simulink model "PubIfDecisionTOS_MDL"  (R2020b)
settings: configuration reference "DspaceConfig" (kept outside this file)
PostLoadFcn:
  | if any(exist('dsrtsu_mdlpostloadfcn', 'file') ~= 0), dsrtsu_mdlpostloadfcn('Execute', bdroot); end
InitFcn:
  | , if any(exist('dsmpb_private', 'file') ~= 0), dsmpb_private('dsmpb_mdlclblib', 'Init', bdroot); end,
undefined symbols (not defined in the file or in its folder): C_TOS_ACCEgoRAxletoFbumplength_m, C_TOS_ACCTargetFront_Flag, C_TOS_AEBJAPedObjDxThre_Val, C_TOS_AEBJAPedObjDyThre_Val, C_TOS_AEBJATargetSize_Val, C_TOS_AEBJAVehObjDxThre_Val, C_TOS_AEBJAVehObjDyThre_Val, C_TOS_AEBJuncPedTargetSize_Val, C_TOS_AEBLatObjDxThre_Val, C_TOS_AEBLatPedDyThre_Val, C_TOS_AEBLatTargetSize_Val, C_TOS_AEBLongTargetInEgoFront_Flag, C_TOS_axAbsGround_Parameter, C_TOS_CameraConfirmedFlag, C_TOS_CNsubjWidth, C_TOS_CurrentLaneCoreMinWidth_Val, C_TOS_CutInProb_Val_Zero, C_TOS_CutOutProb_Val_Zero, C_TOS_D2R_Val, C_TOS_DefaultValueObjectToCenterLine_dy, C_TOS_EgoCarWidth_Val, C_TOS_EgoDxRefPoint_m, C_TOS_EgoRAxletoFbumplength_m, C_TOS_HalfWidthVehicle_Con, C_TOS_HWA_CurrentLaneFlag, C_TOS_HWA_LeftLaneFlag, C_TOS_HWA_MovingDir_Vaild, C_TOS_HWA_MovState_Vaild, C_TOS_HWA_RightLaneFlag, C_TOS_LaneLineCourseErrorFront, C_TOS_LaneLineCourseErrorRear, C_TOS_MotorbikeDefaultWidth_m, C_TOS_NumberOfEffectiveTargets, C_TOS_Obj_Age_Val, C_TOS_Objdx_Constraint_Val, C_TOS_ObjectDefaultWidth_m, C_TOS_ObjInCurrentLane_Val, C_TOS_ObjInCurrentLaneValid, C_TOS_ObjInLeftLaneValid, C_TOS_ObjInRightLaneValid, C_TOS_ObjNotInCurrentLane_Val, C_TOS_ObjNotREElementType, C_TOS_ObjPredictDis_dy_ConstantVal_Zeros, C_TOS_ObjToCenterLine_ConstantVal_Zeros, C_TOS_OFMObjIDInvilad_Val, C_TOS_PIL_LatDisCons_Val_zero, C_TOS_PIL_ObjectCutInFlag_b, C_TOS_PIL_ObjectCutOutFlag_b, C_TOS_PIL_ObjLaneProb_al_Val, C_TOS_PP_ObjFusType_FC_Confirm_b, C_TOS_PP_ObjFusType_FC_FR_Confirm_b, C_TOS_PP_ObjFusType_FR_Confirm_b, C_TOS_RE_80BoolDefault_Val, C_TOS_RE_80Single181Default_Val, C_TOS_RE_80Single255Default_Val, C_TOS_RE_80Uint8Default_Val, C_TOS_RE_D2R, C_TOS_RE_D_180_Val, C_TOS_RE_InvalidObjectID_Val, C_TOS_RE_InvalidTargetChainDir_Val ... (+142)
libraries: simulink x1650, TOS_LIB x361, canfdmsglib x14
(part 2 of 69)

== system PubIfDecisionTOS_MDL/TOS_20201112/TOS_2012080320/Subsystem ==
  TOS_AEBLONOBJ : Inport
  TOS_AEB_JAOBJ : Inport  Port=2
  TOS_AEB_LATOBJ : Inport  Port=3
  Bus Selector : BusSelector  OutputSignals=FusionType,ObjUpdate,ObjectAzimuthAngle,ObjectExistProb,ObjectHight,ObjectID,ObjectIsObstacleProb,ObjectLength,ObjectLengthVar,ObjectLifeCycle,ObjectMeasurementStatus,ObjectMovingOrientationProb,ObjectMovingOrientation,ObjectMovingState,ObjectMovingStateProb,ObjectRCS,ObjectType,ObjectTypeCameraConfirmed,ObjectTypeProb,ObjectWidth,ObjectWidthVar,ObjectYawAngle,ObjectYawAngleVar,ax,axVariance,ay,ayVariance,dx,dxFisrtDetection,dxVariance,dy,dyEgo2Center,dyFisrtDetection,dyObject2Center,dyVariance,dz,vx,vxVariance,vy,vyVariance
  CAN FD Pack : canfdmsglib/CAN FD Pack  CANdbFile=F:\InternalData03_ACC_AEBLog_ELK_LC_LCKie_20200927.dbc  MsgList=(none)  MsgName=TOS_AEBLong  ProtocolMode=CAN FD  MsgIDType=Standard (11-bit identifier)  MsgIdentifier=514  MsgLength=64  Remote=off  BRSSwitch=off  ApplyMinMax=off  SignalInfo={'{'AEBLong_FusionType','24','4','BE','unsigned','Standard','0','1','0','0','15';'AEBLong_ObjUpdate','358','2','BE','unsigned','Standard','0','1','0','0','3';'AEBLong_ObjectAzimuthAngle','231','17','BE','signed','Standard','0','0.0055','0','-360.448','360.4425';'AEBLong_ObjectExistProb','246','10','BE','unsigned','Standard','0','0.000978','0','0','1.0005';'AEBLong_ObjectHight','260','12','BE','unsigned','Standard','0','0.002442','0','0','10';'AEBLong_ObjectID','224','7','BE','unsigned','Standard','0','1','0','0','127';'AEBLong_ObjectIsObstacleProb','278','10','BE','unsigned','Standard','0','0.000978','0','0','1.0005';'AEBLong_ObjectLength','290','14','BE','unsigned','Standard','0','0.0025','0','0','40.9575';'AEBLong_ObjectLengthVar','308','12','BE','unsigned','Standard','0','0.006105','0','0','25';'AEBLong_ObjectLifeCycle','312','8','BE','unsigned','Standard','0','1','0','0','255';'AEBLong_ObjectMeasurementStatus','59','1','BE','unsigned','Standard','0','1','0','0','1';'AEBLong_ObjectMovingOrientProb','334','10','BE','unsigned','Standard','0','0.000978','0','0','1.0005';'AEBLong_ObjectMovingOrientation','104','4','BE','unsigned','Standard','0','1','0','0','15';'AEBLong_ObjectMovingState','120','4','BE','unsigned','Standard','0','1','0','0','15';'AEBLong_ObjectMovingStateProb','350','10','BE','unsigned','Standard','0','0.000978','0','0','1.0005';'AEBLong_ObjectRCS','58','1','BE','unsigned','Standard','0','1','0','0','1';'AEBLong_ObjectType','152','4','BE','unsigned','Standard','0','1','0','0','15';'AEBLong_ObjectTypeCameraConf','57','1','BE','unsigned','Standard','0','1','0','0','1';'AEBLong_ObjectTypeProb','382','10','BE','unsigned','Standard','0','0.000978','0','0','1.0005';'AEBLong_ObjectWidth','396','12','BE','unsigned','Standard','0','0.005','0','0','20.475';'AEBLong_ObjectWidthVar','412','12','BE','unsigned','Standard','0','0.006105','0','0','25';'AEBLong_ObjectYawAngle','439','17','BE','signed','Standard','0','0.0055','0','-360.448','360.4425';'AEBLong_ObjectYawAngleVar','452','12','BE','unsigned','Standard','0','0.006105','0','0','25';'AEBLong_ax','8','16','BE','signed','Standard','0','0.001','0','-32.768','32.767';'AEBLong_axVariance','28','12','BE','unsigned','Standard','0','0.006105','0','0','25';'AEBLong_ay','40','16','BE','signed','Standard','0','0.001','0','-32.768','32.767';'AEBLong_ayVariance','60','12','BE','unsigned','Standard','0','0.006105','0','0','25';'AEBLong_dx','72','16','BE','unsigned','Standard','0','0.0030518','0','0','199.9997';'AEBLong_dxFisrtDetection','88','16','BE','unsigned','Standard','0','0.0030518','0','0','199.9997';'AEBLong_dxVariance','108','12','BE','unsigned','Standard','0','0.006105','0','0','25';'AEBLong_dy','124','12','BE','unsigned','Standard','0','0.009768','0','0','40';'AEBLong_dyEgo2Center','138','14','BE','unsigned','Standard','0','0.0030518','0','0','49.9976';'AEBLong_dyFisrtDetection','156','12','BE','unsigned','Standard','0','0.009768','0','0','40';'AEBLong_dyObject2Center','170','14','BE','unsigned','Standard','0','0.0030518','0','0','49.9976';'AEBLong_dyVariance','188','12','BE','unsigned','Standard','0','0.006105','0','0','25';'AEBLong_dz','204','12','BE','unsigned','Standard','0','0.002442','0','0','10';'AEBLong_vx','472','16','BE','signed','Standard','0','0.006103','0','-199.9831','199.977';'AEBLong_vxVariance','492','12','BE','unsigned','Standard','0','0.006105','0','0','25';'AEBLong_vy','506','14','BE','signed','Standard','0','0.002442','0','-20.0049','20.0024'}
      settings: SourceProductBaseCode=VN  DataFormat=CANdb specified signals
  CAN FD Pack1 : canfdmsglib/CAN FD Pack  CANdbFile=F:\InternalData03_AEB_Lat_JA_20200927.DBC  MsgList=(none)  MsgName=TOS_AEBLarCro_1  ProtocolMode=CAN FD  MsgIDType=Standard (11-bit identifier)  MsgIdentifier=549  MsgLength=64  Remote=off  BRSSwitch=on  ApplyMinMax=off  SignalInfo={'{'AEB_LatCro_FusionType_01','8','7','BE','unsigned','Standard','0','1','0','0','127';'AEB_LatCro_FusionType_02','56','7','BE','unsigned','Standard','0','1','0','0','127';'AEB_LatCro_FusionType_03','96','7','BE','unsigned','Standard','0','1','0','0','127';'AEB_LatCro_FusionType_04','136','7','BE','unsigned','Standard','0','1','0','0','127';'AEB_LatCro_FusionType_05','184','7','BE','unsigned','Standard','0','1','0','0','127';'AEB_LatCro_FusionType_06','224','7','BE','unsigned','Standard','0','1','0','0','127';'AEB_LatCro_FusionType_07','264','7','BE','unsigned','Standard','0','1','0','0','127';'AEB_LatCro_FusionType_08','312','7','BE','unsigned','Standard','0','1','0','0','127';'AEB_LatCro_FusionType_09','352','7','BE','unsigned','Standard','0','1','0','0','127';'AEB_LatCro_FusionType_10','392','7','BE','unsigned','Standard','0','1','0','0','127';'AEB_LatCro_ID_01','24','7','BE','unsigned','Standard','0','1','0','0','127';'AEB_LatCro_ID_02','72','7','BE','unsigned','Standard','0','1','0','0','127';'AEB_LatCro_ID_03','112','7','BE','unsigned','Standard','0','1','0','0','127';'AEB_LatCro_ID_04','152','7','BE','unsigned','Standard','0','1','0','0','127';'AEB_LatCro_ID_05','200','7','BE','unsigned','Standard','0','1','0','0','127';'AEB_LatCro_ID_06','240','7','BE','unsigned','Standard','0','1','0','0','127';'AEB_LatCro_ID_07','280','7','BE','unsigned','Standard','0','1','0','0','127';'AEB_LatCro_ID_08','328','7','BE','unsigned','Standard','0','1','0','0','127';'AEB_LatCro_ID_09','368','7','BE','unsigned','Standard','0','1','0','0','127';'AEB_LatCro_ID_10','408','7','BE','unsigned','Standard','0','1','0','0','127';'AEB_LatCro_MovOrit_01','34','3','BE','unsigned','Standard','0','1','0','0','7';'AEB_LatCro_MovOrit_02','40','3','BE','unsigned','Standard','0','1','0','0','7';'AEB_LatCro_MovOrit_03','125','3','BE','unsigned','Standard','0','1','0','0','7';'AEB_LatCro_MovOrit_04','162','3','BE','unsigned','Standard','0','1','0','0','7';'AEB_LatCro_MovOrit_05','168','3','BE','unsigned','Standard','0','1','0','0','7';'AEB_LatCro_MovOrit_06','253','3','BE','unsigned','Standard','0','1','0','0','7';'AEB_LatCro_MovOrit_07','290','3','BE','unsigned','Standard','0','1','0','0','7';'AEB_LatCro_MovOrit_08','296','3','BE','unsigned','Standard','0','1','0','0','7';'AEB_LatCro_MovOrit_09','381','3','BE','unsigned','Standard','0','1','0','0','7';'AEB_LatCro_MovOrit_10','418','3','BE','unsigned','Standard','0','1','0','0','7';'AEB_LatCro_MovingState_01','37','3','BE','unsigned','Standard','0','1','0','0','7';'AEB_LatCro_MovingState_02','43','3','BE','unsigned','Standard','0','1','0','0','7';'AEB_LatCro_MovingState_03','81','3','BE','unsigned','Standard','0','1','0','0','7';'AEB_LatCro_MovingState_04','165','3','BE','unsigned','Standard','0','1','0','0','7';'AEB_LatCro_MovingState_05','171','3','BE','unsigned','Standard','0','1','0','0','7';'AEB_LatCro_MovingState_06','209','3','BE','unsigned','Standard','0','1','0','0','7';'AEB_LatCro_MovingState_07','293','3','BE','unsigned','Standard','0','1','0','0','7';'AEB_LatCro_MovingState_08','299','3','BE','unsigned','Standard','0','1','0','0','7';'AEB_LatCro_MovingState_09','337','3','BE','unsigned','Standard','0','1','0','0','7';'AEB_LatCro_MovingState_10','421','3','BE','unsigned','Standard','0','1','0','0','7';'AEB_LatCro_ObjectType_01','46','4','BE','unsigned','Standard','0','1','0','0','15';'AEB_LatCro_ObjectType_02','84','4','BE','unsigned','Standard','0','1','0','0','15';'AEB_LatCro_ObjectType_03','121','4','BE','unsigned','Standard','0','1','0','0','15';'AEB_LatCro_ObjectType_04','174','4','BE','unsigned','Standard','0','1','0','0','15';'AEB_LatCro_ObjectType_05','212','4','BE','unsigned','Standard','0','1','0','0','15';'AEB_LatCro_ObjectType_06','249','4','BE','unsigned','Standard','0','1','0','0','15';'AEB_LatCro_ObjectType_07','302','4','BE','unsigned','Standard','0','1','0','0','15';'AEB_LatCro_ObjectType_08','340','4','BE','unsigned','Standard','0','1','0','0','15';'AEB_LatCro_ObjectType_09','377','4','BE','unsigned','Standard','0','1','0','0','15';'AEB_LatCro_ObjectType_10','428','4','BE','unsigned','Standard','0','1','0','0','15';'AEB_LatCro_dx_01','15','9','BE','unsigned','Standard','0','0.1','0','0','51.1';'AEB_LatCro_dx_02','63','9','BE','unsigned','Standard','0','0.1','0','0','51.1';'AEB_LatCro_dx_03','103','9','BE','unsigned','Standard','0','0.1','0','0','51.1';'AEB_LatCro_dx_04','143','9','BE','unsigned','Standard','0','0.1','0','0','51.1';'AEB_LatCro_dx_05','191','9','BE','unsigned','Standard','0','0.1','0','0','51.1';'AEB_LatCro_dx_06','231','9','BE','unsigned','Standard','0','0.1','0','0','51.1';'AEB_LatCro_dx_07','271','9','BE','unsigned','Standard','0','0.1','0','0','51.1';'AEB_LatCro_dx_08','319','9','BE','unsigned','Standard','0','0.1','0','0','51.1';'AEB_LatCro_dx_09','359','9','BE','unsigned','Standard','0','0.1','0','0','51.1';'AEB_LatCro_dx_10','399','9','BE','unsigned','Standard','0','0.1','0','0','51.1';'AEB_LatCro_dy_01','31','9','BE','signed','Standard','0','0.06','0','-15.36','15.3';'AEB_LatCro_dy_02','79','9','BE','signed','Standard','0','0.06','0','-15.36','15.3';'AEB_LatCro_dy_03','119','9','BE','signed','Standard','0','0.06','0','-15.36','15.3';'AEB_LatCro_dy_04','159','9','BE','signed','Standard','0','0.06','0','-15.36','15.3';'AEB_LatCro_dy_05','207','9','BE','signed','Standard','0','0.06','0','-15.36','15.3';'AEB_LatCro_dy_06','247','9','BE','signed','Standard','0','0.06','0','-15.36','15.3';'AEB_LatCro_dy_07','287','9','BE','signed','Standard','0','0.06','0','-15.36','15.3';'AEB_LatCro_dy_08','335','9','BE','signed','Standard','0','0.06','0','-15.36','15.3';'AEB_LatCro_dy_09','375','9','BE','signed','Standard','0','0.06','0','-15.36','15.3'}
      settings: SourceProductBaseCode=VN  DataFormat=CANdb specified signals
  CAN FD Pack2 : canfdmsglib/CAN FD Pack  CANdbFile=F:\InternalData03_AEB_Lat_JA_20200927.DBC  MsgList=(none)  MsgName=TOS_AEB_Junc_1  ProtocolMode=CAN FD  MsgIDType=Standard (11-bit identifier)  MsgIdentifier=545  MsgLength=64  Remote=off  BRSSwitch=on  ApplyMinMax=off  SignalInfo={'{'AEB_Junc_FusionType_01','8','7','BE','unsigned','Standard','0','1','0','0','127';'AEB_Junc_FusionType_02','56','7','BE','unsigned','Standard','0','1','0','0','127';'AEB_Junc_FusionType_03','96','7','BE','unsigned','Standard','0','1','0','0','127';'AEB_Junc_FusionType_04','136','7','BE','unsigned','Standard','0','1','0','0','127';'AEB_Junc_FusionType_05','184','7','BE','unsigned','Standard','0','1','0','0','127';'AEB_Junc_FusionType_06','224','7','BE','unsigned','Standard','0','1','0','0','127';'AEB_Junc_FusionType_07','264','7','BE','unsigned','Standard','0','1','0','0','127';'AEB_Junc_FusionType_08','312','7','BE','unsigned','Standard','0','1','0','0','127';'AEB_Junc_FusionType_09','352','7','BE','unsigned','Standard','0','1','0','0','127';'AEB_Junc_FusionType_10','392','7','BE','unsigned','Standard','0','1','0','0','127';'AEB_Junc_FusionType_11','440','7','BE','unsigned','Standard','0','1','0','0','127';'AEB_Junc_FusionType_12','480','7','BE','unsigned','Standard','0','1','0','0','127';'AEB_Junc_ID_01','24','7','BE','unsigned','Standard','0','1','0','0','127';'AEB_Junc_ID_02','72','7','BE','unsigned','Standard','0','1','0','0','127';'AEB_Junc_ID_03','112','7','BE','unsigned','Standard','0','1','0','0','127';'AEB_Junc_ID_04','152','7','BE','unsigned','Standard','0','1','0','0','127';'AEB_Junc_ID_05','200','7','BE','unsigned','Standard','0','1','0','0','127';'AEB_Junc_ID_06','240','7','BE','unsigned','Standard','0','1','0','0','127';'AEB_Junc_ID_07','280','7','BE','unsigned','Standard','0','1','0','0','127';'AEB_Junc_ID_08','328','7','BE','unsigned','Standard','0','1','0','0','127';'AEB_Junc_ID_09','368','7','BE','unsigned','Standard','0','1','0','0','127';'AEB_Junc_ID_10','408','7','BE','unsigned','Standard','0','1','0','0','127';'AEB_Junc_ID_11','456','7','BE','unsigned','Standard','0','1','0','0','127';'AEB_Junc_ID_12','496','7','BE','unsigned','Standard','0','1','0','0','127';'AEB_Junc_MovOrit_01','34','3','BE','unsigned','Standard','0','1','0','0','7';'AEB_Junc_MovOrit_02','40','3','BE','unsigned','Standard','0','1','0','0','7';'AEB_Junc_MovOrit_03','125','3','BE','unsigned','Standard','0','1','0','0','7';'AEB_Junc_MovOrit_04','162','3','BE','unsigned','Standard','0','1','0','0','7';'AEB_Junc_MovOrit_05','168','3','BE','unsigned','Standard','0','1','0','0','7';'AEB_Junc_MovOrit_06','253','3','BE','unsigned','Standard','0','1','0','0','7';'AEB_Junc_MovOrit_07','290','3','BE','unsigned','Standard','0','1','0','0','7';'AEB_Junc_MovOrit_08','296','3','BE','unsigned','Standard','0','1','0','0','7';'AEB_Junc_MovOrit_09','381','3','BE','unsigned','Standard','0','1','0','0','7';'AEB_Junc_MovOrit_10','418','3','BE','unsigned','Standard','0','1','0','0','7';'AEB_Junc_MovOrit_11','424','3','BE','unsigned','Standard','0','1','0','0','7';'AEB_Junc_MovOrit_12','509','3','BE','unsigned','Standard','0','1','0','0','7';'AEB_Junc_MovingState_01','37','3','BE','unsigned','Standard','0','1','0','0','7';'AEB_Junc_MovingState_02','43','3','BE','unsigned','Standard','0','1','0','0','7';'AEB_Junc_MovingState_03','81','3','BE','unsigned','Standard','0','1','0','0','7';'AEB_Junc_MovingState_04','165','3','BE','unsigned','Standard','0','1','0','0','7';'AEB_Junc_MovingState_05','171','3','BE','unsigned','Standard','0','1','0','0','7';'AEB_Junc_MovingState_06','209','3','BE','unsigned','Standard','0','1','0','0','7';'AEB_Junc_MovingState_07','293','3','BE','unsigned','Standard','0','1','0','0','7';'AEB_Junc_MovingState_08','299','3','BE','unsigned','Standard','0','1','0','0','7';'AEB_Junc_MovingState_09','337','3','BE','unsigned','Standard','0','1','0','0','7';'AEB_Junc_MovingState_10','421','3','BE','unsigned','Standard','0','1','0','0','7';'AEB_Junc_MovingState_11','427','3','BE','unsigned','Standard','0','1','0','0','7';'AEB_Junc_MovingState_12','465','3','BE','unsigned','Standard','0','1','0','0','7';'AEB_Junc_ObjectType_01','46','4','BE','unsigned','Standard','0','1','0','0','15';'AEB_Junc_ObjectType_02','84','4','BE','unsigned','Standard','0','1','0','0','15';'AEB_Junc_ObjectType_03','121','4','BE','unsigned','Standard','0','1','0','0','15';'AEB_Junc_ObjectType_04','174','4','BE','unsigned','Standard','0','1','0','0','15';'AEB_Junc_ObjectType_05','212','4','BE','unsigned','Standard','0','1','0','0','15';'AEB_Junc_ObjectType_06','249','4','BE','unsigned','Standard','0','1','0','0','15';'AEB_Junc_ObjectType_07','302','4','BE','unsigned','Standard','0','1','0','0','15';'AEB_Junc_ObjectType_08','340','4','BE','unsigned','Standard','0','1','0','0','15';'AEB_Junc_ObjectType_09','377','4','BE','unsigned','Standard','0','1','0','0','15';'AEB_Junc_ObjectType_10','430','4','BE','unsigned','Standard','0','1','0','0','15';'AEB_Junc_ObjectType_11','468','4','BE','unsigned','Standard','0','1','0','0','15';'AEB_Junc_ObjectType_12','505','4','BE','unsigned','Standard','0','1','0','0','15';'AEB_Junc_dx_01','15','9','BE','unsigned','Standard','0','0.1','0','0','51.1';'AEB_Junc_dx_02','63','9','BE','unsigned','Standard','0','0.1','0','0','51.1';'AEB_Junc_dx_03','103','9','BE','unsigned','Standard','0','0.1','0','0','51.1';'AEB_Junc_dx_04','143','9','BE','unsigned','Standard','0','0.1','0','0','51.1';'AEB_Junc_dx_05','191','9','BE','unsigned','Standard','0','0.1','0','0','51.1';'AEB_Junc_dx_06','231','9','BE','unsigned','Standard','0','0.1','0','0','51.1';'AEB_Junc_dx_07','271','9','BE','unsigned','Standard','0','0.1','0','0','51.1';'AEB_Junc_dx_08','319','9','BE','unsigned','Standard','0','0.1','0','0','51.1';'AEB_Junc_dx_09','359','9','BE','unsigned','Standard','0','0.1','0','0','51.1';'AEB_Junc_dx_10','399','9','BE','unsigned','Standard','0','0.1','0','0','51.1';'AEB_Junc_dx_11','447','9','BE','unsigned','Standard','0','0.1','0','0','51.1';'AEB_Junc_dx_12','487','9','BE','unsigned','Standard','0','0.1','0','0','51.1';'AEB_Junc_dy_01','31','9','BE','signed','Standard','0','0.06','0','-15.36','15.3';'AEB_Junc_dy_02','79','9','BE','signed','Standard','0','0.06','0','-15.36','15.3';'AEB_Junc_dy_03','119','9','BE','signed','Standard','0','0.06','0','-15.36','15.3';'AEB_Junc_dy_04','159','9','BE','signed','Standard','0','0.06','0','-15.36','15.3';'AEB_Junc_dy_05','207','9','BE','signed','Standard','0','0.06','0','-15.36','15.3';'AEB_Junc_dy_06','247','9','BE','signed','Standard','0','0.06','0','-15.36','15.3';'AEB_Junc_dy_07','287','9','BE','signed','Standard','0','0.06','0','-15.36','15.3';'AEB_Junc_dy_08','335','9','BE','signed','Standard','0','0.06','0','-15.36','15.3';'AEB_Junc_dy_09','375','9','BE','signed','Standard','0','0.06','0','-15.36','15.3';'AEB_Junc_dy_10','415','9','BE','signed','Standard','0','0.06','0','-15.36','15.3';'AEB_Junc_dy_11','463','9','BE','signed','Standard','0','0.06','0','-15.36','15.3'}
      settings: SourceProductBaseCode=VN  DataFormat=CANdb specified signals
  CAN FD Pack3 : canfdmsglib/CAN FD Pack  CANdbFile=F:\InternalData03_AEB_Lat_JA_20200927.DBC  MsgList=(none)  MsgName=TOS_AEB_Junc_2  ProtocolMode=CAN FD  MsgIDType=Standard (11-bit identifier)  MsgIdentifier=546  MsgLength=64  Remote=off  BRSSwitch=on  ApplyMinMax=off  SignalInfo={'{'AEB_Junc_FusionType_13','8','7','BE','unsigned','Standard','0','1','0','0','127';'AEB_Junc_FusionType_14','56','7','BE','unsigned','Standard','0','1','0','0','127';'AEB_Junc_FusionType_15','96','7','BE','unsigned','Standard','0','1','0','0','127';'AEB_Junc_FusionType_16','136','7','BE','unsigned','Standard','0','1','0','0','127';'AEB_Junc_FusionType_17','184','7','BE','unsigned','Standard','0','1','0','0','127';'AEB_Junc_FusionType_18','224','7','BE','unsigned','Standard','0','1','0','0','127';'AEB_Junc_FusionType_19','264','7','BE','unsigned','Standard','0','1','0','0','127';'AEB_Junc_FusionType_20','312','7','BE','unsigned','Standard','0','1','0','0','127';'AEB_Junc_FusionType_21','352','7','BE','unsigned','Standard','0','1','0','0','127';'AEB_Junc_FusionType_22','392','7','BE','unsigned','Standard','0','1','0','0','127';'AEB_Junc_FusionType_23','440','7','BE','unsigned','Standard','0','1','0','0','127';'AEB_Junc_FusionType_24','480','7','BE','unsigned','Standard','0','1','0','0','127';'AEB_Junc_ID_13','24','7','BE','unsigned','Standard','0','1','0','0','127';'AEB_Junc_ID_14','72','7','BE','unsigned','Standard','0','1','0','0','127';'AEB_Junc_ID_15','112','7','BE','unsigned','Standard','0','1','0','0','127';'AEB_Junc_ID_16','152','7','BE','unsigned','Standard','0','1','0','0','127';'AEB_Junc_ID_17','200','7','BE','unsigned','Standard','0','1','0','0','127';'AEB_Junc_ID_18','240','7','BE','unsigned','Standard','0','1','0','0','127';'AEB_Junc_ID_19','280','7','BE','unsigned','Standard','0','1','0','0','127';'AEB_Junc_ID_20','328','7','BE','unsigned','Standard','0','1','0','0','127';'AEB_Junc_ID_21','368','7','BE','unsigned','Standard','0','1','0','0','127';'AEB_Junc_ID_22','408','7','BE','unsigned','Standard','0','1','0','0','127';'AEB_Junc_ID_23','456','7','BE','unsigned','Standard','0','1','0','0','127';'AEB_Junc_ID_24','496','7','BE','unsigned','Standard','0','1','0','0','127';'AEB_Junc_MovOrit_13','34','3','BE','unsigned','Standard','0','1','0','0','7';'AEB_Junc_MovOrit_14','40','3','BE','unsigned','Standard','0','1','0','0','7';'AEB_Junc_MovOrit_15','125','3','BE','unsigned','Standard','0','1','0','0','7';'AEB_Junc_MovOrit_16','162','3','BE','unsigned','Standard','0','1','0','0','7';'AEB_Junc_MovOrit_17','168','3','BE','unsigned','Standard','0','1','0','0','7';'AEB_Junc_MovOrit_18','253','3','BE','unsigned','Standard','0','1','0','0','7';'AEB_Junc_MovOrit_19','290','3','BE','unsigned','Standard','0','1','0','0','7';'AEB_Junc_MovOrit_20','296','3','BE','unsigned','Standard','0','1','0','0','7';'AEB_Junc_MovOrit_21','381','3','BE','unsigned','Standard','0','1','0','0','7';'AEB_Junc_MovOrit_22','418','3','BE','unsigned','Standard','0','1','0','0','7';'AEB_Junc_MovOrit_23','424','3','BE','unsigned','Standard','0','1','0','0','7';'AEB_Junc_MovOrit_24','509','3','BE','unsigned','Standard','0','1','0','0','7';'AEB_Junc_MovingState_13','37','3','BE','unsigned','Standard','0','1','0','0','7';'AEB_Junc_MovingState_14','43','3','BE','unsigned','Standard','0','1','0','0','7';'AEB_Junc_MovingState_15','81','3','BE','unsigned','Standard','0','1','0','0','7';'AEB_Junc_MovingState_16','165','3','BE','unsigned','Standard','0','1','0','0','7';'AEB_Junc_MovingState_17','171','3','BE','unsigned','Standard','0','1','0','0','7';'AEB_Junc_MovingState_18','209','3','BE','unsigned','Standard','0','1','0','0','7';'AEB_Junc_MovingState_19','293','3','BE','unsigned','Standard','0','1','0','0','7';'AEB_Junc_MovingState_20','299','3','BE','unsigned','Standard','0','1','0','0','7';'AEB_Junc_MovingState_21','337','3','BE','unsigned','Standard','0','1','0','0','7';'AEB_Junc_MovingState_22','421','3','BE','unsigned','Standard','0','1','0','0','7';'AEB_Junc_MovingState_23','427','3','BE','unsigned','Standard','0','1','0','0','7';'AEB_Junc_MovingState_24','465','3','BE','unsigned','Standard','0','1','0','0','7';'AEB_Junc_ObjectType_13','46','4','BE','unsigned','Standard','0','1','0','0','15';'AEB_Junc_ObjectType_14','84','4','BE','unsigned','Standard','0','1','0','0','15';'AEB_Junc_ObjectType_15','121','4','BE','unsigned','Standard','0','1','0','0','15';'AEB_Junc_ObjectType_16','174','4','BE','unsigned','Standard','0','1','0','0','15';'AEB_Junc_ObjectType_17','212','4','BE','unsigned','Standard','0','1','0','0','15';'AEB_Junc_ObjectType_18','249','4','BE','unsigned','Standard','0','1','0','0','15';'AEB_Junc_ObjectType_19','302','4','BE','unsigned','Standard','0','1','0','0','15';'AEB_Junc_ObjectType_20','340','4','BE','unsigned','Standard','0','1','0','0','15';'AEB_Junc_ObjectType_21','377','4','BE','unsigned','Standard','0','1','0','0','15';'AEB_Junc_ObjectType_22','430','4','BE','unsigned','Standard','0','1','0','0','15';'AEB_Junc_ObjectType_23','468','4','BE','unsigned','Standard','0','1','0','0','15';'AEB_Junc_ObjectType_24','505','4','BE','unsigned','Standard','0','1','0','0','15';'AEB_Junc_dx_13','15','9','BE','unsigned','Standard','0','0.1','0','0','51.1';'AEB_Junc_dx_14','63','9','BE','unsigned','Standard','0','0.1','0','0','51.1';'AEB_Junc_dx_15','103','9','BE','unsigned','Standard','0','0.1','0','0','51.1';'AEB_Junc_dx_16','143','9','BE','unsigned','Standard','0','0.1','0','0','51.1';'AEB_Junc_dx_17','191','9','BE','unsigned','Standard','0','0.1','0','0','51.1';'AEB_Junc_dx_18','231','9','BE','unsigned','Standard','0','0.1','0','0','51.1';'AEB_Junc_dx_19','271','9','BE','unsigned','Standard','0','0.1','0','0','51.1';'AEB_Junc_dx_20','319','9','BE','unsigned','Standard','0','0.1','0','0','51.1';'AEB_Junc_dx_21','359','9','BE','unsigned','Standard','0','0.1','0','0','51.1';'AEB_Junc_dx_22','399','9','BE','unsigned','Standard','0','0.1','0','0','51.1';'AEB_Junc_dx_23','447','9','BE','unsigned','Standard','0','0.1','0','0','51.1';'AEB_Junc_dx_24','487','9','BE','unsigned','Standard','0','0.1','0','0','51.1';'AEB_Junc_dy_13','31','9','BE','signed','Standard','0','0.06','0','-15.36','15.3';'AEB_Junc_dy_14','79','9','BE','signed','Standard','0','0.06','0','-15.36','15.3';'AEB_Junc_dy_15','119','9','BE','signed','Standard','0','0.06','0','-15.36','15.3';'AEB_Junc_dy_16','159','9','BE','signed','Standard','0','0.06','0','-15.36','15.3';'AEB_Junc_dy_17','207','9','BE','signed','Standard','0','0.06','0','-15.36','15.3';'AEB_Junc_dy_18','247','9','BE','signed','Standard','0','0.06','0','-15.36','15.3';'AEB_Junc_dy_19','287','9','BE','signed','Standard','0','0.06','0','-15.36','15.3';'AEB_Junc_dy_20','335','9','BE','signed','Standard','0','0.06','0','-15.36','15.3';'AEB_Junc_dy_21','375','9','BE','signed','Standard','0','0.06','0','-15.36','15.3';'AEB_Junc_dy_22','415','9','BE','signed','Standard','0','0.06','0','-15.36','15.3';'AEB_Junc_dy_23','463','9','BE','signed','Standard','0','0.06','0','-15.36','15.3'}
      settings: SourceProductBaseCode=VN  DataFormat=CANdb specified signals
  CAN FD Pack4 : canfdmsglib/CAN FD Pack  CANdbFile=F:\InternalData03_AEB_Lat_JA_20200927.DBC  MsgList=(none)  MsgName=TOS_AEB_Junc_3  ProtocolMode=CAN FD  MsgIDType=Standard (11-bit identifier)  MsgIdentifier=547  MsgLength=64  Remote=off  BRSSwitch=on  ApplyMinMax=off  SignalInfo={'{'AEB_Junc_FusionType_25','8','7','BE','unsigned','Standard','0','1','0','0','127';'AEB_Junc_FusionType_26','56','7','BE','unsigned','Standard','0','1','0','0','127';'AEB_Junc_FusionType_27','96','7','BE','unsigned','Standard','0','1','0','0','127';'AEB_Junc_FusionType_28','136','7','BE','unsigned','Standard','0','1','0','0','127';'AEB_Junc_FusionType_29','184','7','BE','unsigned','Standard','0','1','0','0','127';'AEB_Junc_FusionType_30','224','7','BE','unsigned','Standard','0','1','0','0','127';'AEB_Junc_FusionType_31','264','7','BE','unsigned','Standard','0','1','0','0','127';'AEB_Junc_FusionType_32','312','7','BE','unsigned','Standard','0','1','0','0','127';'AEB_Junc_ID_25','24','7','BE','unsigned','Standard','0','1','0','0','127';'AEB_Junc_ID_26','72','7','BE','unsigned','Standard','0','1','0','0','127';'AEB_Junc_ID_27','112','7','BE','unsigned','Standard','0','1','0','0','127';'AEB_Junc_ID_28','152','7','BE','unsigned','Standard','0','1','0','0','127';'AEB_Junc_ID_29','200','7','BE','unsigned','Standard','0','1','0','0','127';'AEB_Junc_ID_30','240','7','BE','unsigned','Standard','0','1','0','0','127';'AEB_Junc_ID_31','280','7','BE','unsigned','Standard','0','1','0','0','127';'AEB_Junc_ID_32','328','7','BE','unsigned','Standard','0','1','0','0','127';'AEB_Junc_MovOrit_25','34','3','BE','unsigned','Standard','0','1','0','0','7';'AEB_Junc_MovOrit_26','40','3','BE','unsigned','Standard','0','1','0','0','7';'AEB_Junc_MovOrit_27','125','3','BE','unsigned','Standard','0','1','0','0','7';'AEB_Junc_MovOrit_28','162','3','BE','unsigned','Standard','0','1','0','0','7';'AEB_Junc_MovOrit_29','168','3','BE','unsigned','Standard','0','1','0','0','7';'AEB_Junc_MovOrit_30','253','3','BE','unsigned','Standard','0','1','0','0','7';'AEB_Junc_MovOrit_31','290','3','BE','unsigned','Standard','0','1','0','0','7';'AEB_Junc_MovOrit_32','296','3','BE','unsigned','Standard','0','1','0','0','7';'AEB_Junc_MovingState_25','37','3','BE','unsigned','Standard','0','1','0','0','7';'AEB_Junc_MovingState_26','43','3','BE','unsigned','Standard','0','1','0','0','7';'AEB_Junc_MovingState_27','81','3','BE','unsigned','Standard','0','1','0','0','7';'AEB_Junc_MovingState_28','165','3','BE','unsigned','Standard','0','1','0','0','7';'AEB_Junc_MovingState_29','171','3','BE','unsigned','Standard','0','1','0','0','7';'AEB_Junc_MovingState_30','209','3','BE','unsigned','Standard','0','1','0','0','7';'AEB_Junc_MovingState_31','293','3','BE','unsigned','Standard','0','1','0','0','7';'AEB_Junc_MovingState_32','299','3','BE','unsigned','Standard','0','1','0','0','7';'AEB_Junc_ObjectType_25','46','4','BE','unsigned','Standard','0','1','0','0','15';'AEB_Junc_ObjectType_26','84','4','BE','unsigned','Standard','0','1','0','0','15';'AEB_Junc_ObjectType_27','121','4','BE','unsigned','Standard','0','1','0','0','15';'AEB_Junc_ObjectType_28','174','4','BE','unsigned','Standard','0','1','0','0','15';'AEB_Junc_ObjectType_29','212','4','BE','unsigned','Standard','0','1','0','0','15';'AEB_Junc_ObjectType_30','249','4','BE','unsigned','Standard','0','1','0','0','15';'AEB_Junc_ObjectType_31','302','4','BE','unsigned','Standard','0','1','0','0','15';'AEB_Junc_ObjectType_32','340','4','BE','unsigned','Standard','0','1','0','0','15';'AEB_Junc_dx_25','15','9','BE','unsigned','Standard','0','0.1','0','0','51.1';'AEB_Junc_dx_26','63','9','BE','unsigned','Standard','0','0.1','0','0','51.1';'AEB_Junc_dx_27','103','9','BE','unsigned','Standard','0','0.1','0','0','51.1';'AEB_Junc_dx_28','143','9','BE','unsigned','Standard','0','0.1','0','0','51.1';'AEB_Junc_dx_29','191','9','BE','unsigned','Standard','0','0.1','0','0','51.1';'AEB_Junc_dx_30','231','9','BE','unsigned','Standard','0','0.1','0','0','51.1';'AEB_Junc_dx_31','271','9','BE','unsigned','Standard','0','0.1','0','0','51.1';'AEB_Junc_dx_32','319','9','BE','unsigned','Standard','0','0.1','0','0','51.1';'AEB_Junc_dy_25','31','9','BE','signed','Standard','0','0.06','0','-15.36','15.3';'AEB_Junc_dy_26','79','9','BE','signed','Standard','0','0.06','0','-15.36','15.3';'AEB_Junc_dy_27','119','9','BE','signed','Standard','0','0.06','0','-15.36','15.3';'AEB_Junc_dy_28','159','9','BE','signed','Standard','0','0.06','0','-15.36','15.3';'AEB_Junc_dy_29','207','9','BE','signed','Standard','0','0.06','0','-15.36','15.3';'AEB_Junc_dy_30','247','9','BE','signed','Standard','0','0.06','0','-15.36','15.3';'AEB_Junc_dy_31','287','9','BE','signed','Standard','0','0.06','0','-15.36','15.3'}
      settings: SourceProductBaseCode=VN  DataFormat=CANdb specified signals
  Demux{1..6,28} (7 alike) : Demux  Outputs=10
  Demux{7..20} (14 alike) : Demux  Outputs=12
  Demux{21..27} (7 alike) : Demux  Outputs=8
  For Each Subsystem : Subsystem  TreatAsAtomicUnit=on
  For Each Subsystem1 : Subsystem  TreatAsAtomicUnit=on
  Selector{,1..6} (7 alike) : Selector  InputPortWidth=32  IndexOptions=Index vector (dialog)  Indices=[1:12]  OutputSizes=1
  Selector{7..13} (7 alike) : Selector  InputPortWidth=32  IndexOptions=Index vector (dialog)  Indices=[13:24]  OutputSizes=1
  Selector{14..20} (7 alike) : Selector  InputPortWidth=32  IndexOptions=Index vector (dialog)  Indices=[25:32]  OutputSizes=1
  TOS_AEBLONOBJ_Msg : Outport
  TOS_AEB_JAOBJ1_Msg : Outport  Port=2
  TOS_AEB_LATOBJ_Msg : Outport  Port=3
  TOS_AEB_JAOBJ2_Msg : Outport  Port=4
  TOS_AEB_JAOBJ3_Msg : Outport  Port=5
  wires:
  CAN FD Pack/1 -> TOS_AEBLONOBJ_Msg/1
  TOS_AEBLONOBJ/1 -> Bus Selector/1
  Bus Selector/1 -> CAN FD Pack/1  "<FusionType>"
  Bus Selector/2 -> CAN FD Pack/2  "<ObjUpdate>"
  Bus Selector/3 -> CAN FD Pack/3  "<ObjectAzimuthAngle>"
  Bus Selector/4 -> CAN FD Pack/4  "<ObjectExistProb>"
  Bus Selector/5 -> CAN FD Pack/5  "<ObjectHight>"
  Bus Selector/6 -> CAN FD Pack/6  "<ObjectID>"
  Bus Selector/7 -> CAN FD Pack/7  "<ObjectIsObstacleProb>"
  Bus Selector/8 -> CAN FD Pack/8  "<ObjectLength>"
  Bus Selector/9 -> CAN FD Pack/9  "<ObjectLengthVar>"
  Bus Selector/10 -> CAN FD Pack/10  "<ObjectLifeCycle>"
  Bus Selector/11 -> CAN FD Pack/11  "<ObjectMeasurementStatus>"
  Bus Selector/12 -> CAN FD Pack/12  "<ObjectMovingOrientationProb>"
  Bus Selector/13 -> CAN FD Pack/13  "<ObjectMovingOrientation>"
  Bus Selector/14 -> CAN FD Pack/14  "<ObjectMovingState>"
  Bus Selector/15 -> CAN FD Pack/15  "<ObjectMovingStateProb>"
  Bus Selector/16 -> CAN FD Pack/16  "<ObjectRCS>"
  Bus Selector/17 -> CAN FD Pack/17  "<ObjectType>"
  Bus Selector/18 -> CAN FD Pack/18  "<ObjectTypeCameraConfirmed>"
  Bus Selector/19 -> CAN FD Pack/19  "<ObjectTypeProb>"
  Bus Selector/20 -> CAN FD Pack/20  "<ObjectWidth>"
  Bus Selector/21 -> CAN FD Pack/21  "<ObjectWidthVar>"
  Bus Selector/22 -> CAN FD Pack/22  "<ObjectYawAngle>"
  Bus Selector/23 -> CAN FD Pack/23  "<ObjectYawAngleVar>"
  Bus Selector/24 -> CAN FD Pack/24  "<ax>"
  Bus Selector/25 -> CAN FD Pack/25  "<axVariance>"
  Bus Selector/26 -> CAN FD Pack/26  "<ay>"
  Bus Selector/27 -> CAN FD Pack/27  "<ayVariance>"
  Bus Selector/28 -> CAN FD Pack/28  "<dx>"
  Bus Selector/29 -> CAN FD Pack/29  "<dxFisrtDetection>"
  Bus Selector/30 -> CAN FD Pack/30  "<dxVariance>"
  Bus Selector/31 -> CAN FD Pack/31  "<dy>"
  Bus Selector/32 -> CAN FD Pack/32  "<dyEgo2Center>"
  Bus Selector/33 -> CAN FD Pack/33  "<dyFisrtDetection>"
  Bus Selector/34 -> CAN FD Pack/34  "<dyObject2Center>"
  Bus Selector/35 -> CAN FD Pack/35  "<dyVariance>"
  Bus Selector/36 -> CAN FD Pack/36  "<dz>"
  Bus Selector/37 -> CAN FD Pack/37  "<vx>"
  Bus Selector/38 -> CAN FD Pack/38  "<vxVariance>"
  Bus Selector/39 -> CAN FD Pack/39  "<vy>"
  Bus Selector/40 -> CAN FD Pack/40  "<vyVariance>"
  CAN FD Pack1/1 -> TOS_AEB_LATOBJ_Msg/1
  CAN FD Pack2/1 -> TOS_AEB_JAOBJ1_Msg/1
  Demux7/12 -> CAN FD Pack2/12
  Demux7/11 -> CAN FD Pack2/11
  Demux7/10 -> CAN FD Pack2/10
  Demux7/9 -> CAN FD Pack2/9
  Demux7/8 -> CAN FD Pack2/8
  Demux7/7 -> CAN FD Pack2/7
  Demux7/6 -> CAN FD Pack2/6
  Demux7/5 -> CAN FD Pack2/5
  Demux7/4 -> CAN FD Pack2/4
  Demux7/3 -> CAN FD Pack2/3
  Demux7/2 -> CAN FD Pack2/2
  Demux7/1 -> CAN FD Pack2/1
  Demux8/1 -> CAN FD Pack2/13
  Demux8/2 -> CAN FD Pack2/14
  Demux8/3 -> CAN FD Pack2/15
  Demux8/4 -> CAN FD Pack2/16
  Demux8/5 -> CAN FD Pack2/17
  Demux8/6 -> CAN FD Pack2/18
  Demux8/7 -> CAN FD Pack2/19
  Demux8/8 -> CAN FD Pack2/20
  Demux8/9 -> CAN FD Pack2/21
  Demux8/10 -> CAN FD Pack2/22
  Demux8/11 -> CAN FD Pack2/23
  Demux8/12 -> CAN FD Pack2/24
  Demux10/12 -> CAN FD Pack2/48
  Demux10/11 -> CAN FD Pack2/47
  Demux10/10 -> CAN FD Pack2/46
  Demux10/9 -> CAN FD Pack2/45
  Demux10/8 -> CAN FD Pack2/44
  Demux10/7 -> CAN FD Pack2/43
  Demux10/6 -> CAN FD Pack2/42
  Demux10/5 -> CAN FD Pack2/41
  Demux10/4 -> CAN FD Pack2/40
  Demux10/3 -> CAN FD Pack2/39
  Demux10/2 -> CAN FD Pack2/38
  Demux10/1 -> CAN FD Pack2/37
  Demux9/1 -> CAN FD Pack2/25
  Demux9/2 -> CAN FD Pack2/26
  Demux9/3 -> CAN FD Pack2/27
  Demux9/4 -> CAN FD Pack2/28
  Demux9/5 -> CAN FD Pack2/29
  Demux9/6 -> CAN FD Pack2/30
  Demux9/7 -> CAN FD Pack2/31
  Demux9/8 -> CAN FD Pack2/32
  Demux9/9 -> CAN FD Pack2/33
  Demux9/10 -> CAN FD Pack2/34
  Demux9/11 -> CAN FD Pack2/35
  Demux9/12 -> CAN FD Pack2/36
  Demux12/12 -> CAN FD Pack2/60
  Demux12/11 -> CAN FD Pack2/59
  Demux12/10 -> CAN FD Pack2/58
  Demux12/9 -> CAN FD Pack2/57
  Demux12/8 -> CAN FD Pack2/56
  Demux12/7 -> CAN FD Pack2/55
  Demux12/6 -> CAN FD Pack2/54
  Demux12/5 -> CAN FD Pack2/53
  Demux12/4 -> CAN FD Pack2/52
  Demux12/3 -> CAN FD Pack2/51
  Demux12/2 -> CAN FD Pack2/50
  Demux12/1 -> CAN FD Pack2/49
  Demux11/1 -> CAN FD Pack2/61
  Demux11/2 -> CAN FD Pack2/62
  Demux11/3 -> CAN FD Pack2/63
  Demux11/4 -> CAN FD Pack2/64
  Demux11/5 -> CAN FD Pack2/65
  Demux11/6 -> CAN FD Pack2/66
  Demux11/7 -> CAN FD Pack2/67
  Demux11/8 -> CAN FD Pack2/68
  Demux11/9 -> CAN FD Pack2/69
  Demux11/10 -> CAN FD Pack2/70
  Demux11/11 -> CAN FD Pack2/71
  Demux11/12 -> CAN FD Pack2/72
  Demux13/1 -> CAN FD Pack2/73
  Demux13/2 -> CAN FD Pack2/74
  Demux13/3 -> CAN FD Pack2/75
  Demux13/4 -> CAN FD Pack2/76
  Demux13/5 -> CAN FD Pack2/77
  Demux13/6 -> CAN FD Pack2/78
  Demux13/7 -> CAN FD Pack2/79
  Demux13/8 -> CAN FD Pack2/80
  Demux13/9 -> CAN FD Pack2/81
  Demux13/10 -> CAN FD Pack2/82
  Demux13/11 -> CAN FD Pack2/83
  Demux13/12 -> CAN FD Pack2/84
  Demux17/12 -> CAN FD Pack3/84
  Demux17/11 -> CAN FD Pack3/83
  Demux17/10 -> CAN FD Pack3/82
  Demux17/9 -> CAN FD Pack3/81
  Demux17/8 -> CAN FD Pack3/80
  Demux17/7 -> CAN FD Pack3/79
  Demux17/6 -> CAN FD Pack3/78
  Demux17/5 -> CAN FD Pack3/77
  Demux17/4 -> CAN FD Pack3/76
  Demux17/3 -> CAN FD Pack3/75
  Demux17/2 -> CAN FD Pack3/74
  Demux17/1 -> CAN FD Pack3/73
  Demux15/12 -> CAN FD Pack3/72
  Demux15/11 -> CAN FD Pack3/71
  Demux15/10 -> CAN FD Pack3/70
  Demux15/9 -> CAN FD Pack3/69
  Demux15/8 -> CAN FD Pack3/68
  Demux15/7 -> CAN FD Pack3/67
  Demux15/6 -> CAN FD Pack3/66
  Demux15/5 -> CAN FD Pack3/65
  Demux15/4 -> CAN FD Pack3/64
  Demux15/3 -> CAN FD Pack3/63
  Demux15/2 -> CAN FD Pack3/62
  Demux15/1 -> CAN FD Pack3/61
  Demux16/1 -> CAN FD Pack3/49
  Demux16/2 -> CAN FD Pack3/50
  Demux16/3 -> CAN FD Pack3/51
  Demux16/4 -> CAN FD Pack3/52
  Demux16/5 -> CAN FD Pack3/53
  Demux16/6 -> CAN FD Pack3/54
  Demux16/7 -> CAN FD Pack3/55
  Demux16/8 -> CAN FD Pack3/56
  Demux16/9 -> CAN FD Pack3/57
  Demux16/10 -> CAN FD Pack3/58
  Demux16/11 -> CAN FD Pack3/59
  Demux16/12 -> CAN FD Pack3/60
  Demux20/12 -> CAN FD Pack3/36
  Demux20/11 -> CAN FD Pack3/35
  Demux20/10 -> CAN FD Pack3/34
  Demux20/9 -> CAN FD Pack3/33
  Demux20/8 -> CAN FD Pack3/32
  Demux20/7 -> CAN FD Pack3/31
  Demux20/6 -> CAN FD Pack3/30
  Demux20/5 -> CAN FD Pack3/29
  Demux20/4 -> CAN FD Pack3/28
  Demux20/3 -> CAN FD Pack3/27
  Demux20/2 -> CAN FD Pack3/26
  Demux20/1 -> CAN FD Pack3/25
  Demux14/1 -> CAN FD Pack3/37
  Demux14/2 -> CAN FD Pack3/38
  Demux14/3 -> CAN FD Pack3/39
  Demux14/4 -> CAN FD Pack3/40
  Demux14/5 -> CAN FD Pack3/41
  Demux14/6 -> CAN FD Pack3/42
  Demux14/7 -> CAN FD Pack3/43
  Demux14/8 -> CAN FD Pack3/44
  Demux14/9 -> CAN FD Pack3/45
  Demux14/10 -> CAN FD Pack3/46
  Demux14/11 -> CAN FD Pack3/47
  Demux14/12 -> CAN FD Pack3/48
  Demux19/12 -> CAN FD Pack3/24
  Demux19/11 -> CAN FD Pack3/23
  Demux19/10 -> CAN FD Pack3/22
  Demux19/9 -> CAN FD Pack3/21
  Demux19/8 -> CAN FD Pack3/20
  Demux19/7 -> CAN FD Pack3/19
  Demux19/6 -> CAN FD Pack3/18
  Demux19/5 -> CAN FD Pack3/17
  Demux19/4 -> CAN FD Pack3/16
  Demux19/3 -> CAN FD Pack3/15
  Demux19/2 -> CAN FD Pack3/14
  Demux19/1 -> CAN FD Pack3/13
  Demux18/1 -> CAN FD Pack3/1
  Demux18/2 -> CAN FD Pack3/2
  Demux18/3 -> CAN FD Pack3/3
  Demux18/4 -> CAN FD Pack3/4
  Demux18/5 -> CAN FD Pack3/5
  Demux18/6 -> CAN FD Pack3/6
  Demux18/7 -> CAN FD Pack3/7
  Demux18/8 -> CAN FD Pack3/8
  Demux18/9 -> CAN FD Pack3/9
  Demux18/10 -> CAN FD Pack3/10
  Demux18/11 -> CAN FD Pack3/11
  Demux18/12 -> CAN FD Pack3/12
  Selector/1 -> Demux7/1
  Selector1/1 -> Demux8/1
  Selector2/1 -> Demux9/1
  Selector3/1 -> Demux10/1
  Selector4/1 -> Demux12/1
  Selector5/1 -> Demux11/1
  Selector6/1 -> Demux13/1
  Selector7/1 -> Demux18/1
  Selector8/1 -> Demux19/1
  Selector9/1 -> Demux20/1
  Selector10/1 -> Demux14/1
  Selector11/1 -> Demux16/1
  Selector12/1 -> Demux15/1
  Selector13/1 -> Demux17/1
  Selector20/1 -> Demux26/1
  Selector19/1 -> Demux27/1
  Selector17/1 -> Demux24/1
  Selector16/1 -> Demux22/1
  Selector15/1 -> Demux23/1
  Selector14/1 -> Demux21/1
  Selector18/1 -> Demux25/1
  TOS_AEB_JAOBJ/1 -> For Each Subsystem1/1(In1)
  For Each Subsystem1/1(FusionType) -> Selector18/1, Selector7/1, Selector/1
  For Each Subsystem1/2(ObjectID) -> Selector14/1, Selector8/1, Selector1/1
  For Each Subsystem1/3(ObjectMovingOrientation) -> Selector2/1, Selector15/1, Selector9/1
  For Each Subsystem1/4(ObjectMovingState) -> Selector16/1, Selector10/1, Selector3/1
  For Each Subsystem1/5(ObjectType) -> Selector17/1, Selector11/1, Selector4/1
  For Each Subsystem1/6(dx) -> Selector12/1, Selector19/1, Selector5/1
  For Each Subsystem1/7(dy) -> Selector20/1, Selector13/1, Selector6/1
  CAN FD Pack3/1 -> TOS_AEB_JAOBJ2_Msg/1
  CAN FD Pack4/1 -> TOS_AEB_JAOBJ3_Msg/1
  Demux25/1 -> CAN FD Pack4/1
  Demux25/2 -> CAN FD Pack4/2
  Demux25/3 -> CAN FD Pack4/3
  Demux25/4 -> CAN FD Pack4/4
  Demux25/5 -> CAN FD Pack4/5
  Demux25/6 -> CAN FD Pack4/6
  Demux25/7 -> CAN FD Pack4/7
  Demux25/8 -> CAN FD Pack4/8
  Demux21/1 -> CAN FD Pack4/9
  Demux21/2 -> CAN FD Pack4/10
  Demux21/3 -> CAN FD Pack4/11
  Demux21/4 -> CAN FD Pack4/12
  Demux21/5 -> CAN FD Pack4/13
  Demux21/6 -> CAN FD Pack4/14
  Demux21/7 -> CAN FD Pack4/15
  Demux21/8 -> CAN FD Pack4/16
  Demux22/8 -> CAN FD Pack4/32
  Demux22/7 -> CAN FD Pack4/31
  Demux22/6 -> CAN FD Pack4/30
  Demux22/5 -> CAN FD Pack4/29
  Demux22/4 -> CAN FD Pack4/28
  Demux22/3 -> CAN FD Pack4/27
  Demux22/2 -> CAN FD Pack4/26
  Demux22/1 -> CAN FD Pack4/25
  Demux23/8 -> CAN FD Pack4/24
  Demux23/7 -> CAN FD Pack4/23
  Demux23/6 -> CAN FD Pack4/22
  Demux23/5 -> CAN FD Pack4/21
  Demux23/4 -> CAN FD Pack4/20
  Demux23/3 -> CAN FD Pack4/19
  Demux23/2 -> CAN FD Pack4/18
  Demux23/1 -> CAN FD Pack4/17
  Demux27/1 -> CAN FD Pack4/41
  Demux27/2 -> CAN FD Pack4/42
  Demux27/3 -> CAN FD Pack4/43
  Demux27/4 -> CAN FD Pack4/44
  Demux27/5 -> CAN FD Pack4/45
  Demux27/6 -> CAN FD Pack4/46
  Demux27/7 -> CAN FD Pack4/47
  Demux27/8 -> CAN FD Pack4/48
  Demux26/1 -> CAN FD Pack4/49
  Demux26/2 -> CAN FD Pack4/50
  Demux26/3 -> CAN FD Pack4/51
  Demux26/4 -> CAN FD Pack4/52
  Demux26/5 -> CAN FD Pack4/53
  Demux26/6 -> CAN FD Pack4/54
  Demux26/7 -> CAN FD Pack4/55
  Demux26/8 -> CAN FD Pack4/56
  Demux24/8 -> CAN FD Pack4/40
  Demux24/7 -> CAN FD Pack4/39
  Demux24/6 -> CAN FD Pack4/38
  Demux24/5 -> CAN FD Pack4/37
  Demux24/4 -> CAN FD Pack4/36
  Demux24/3 -> CAN FD Pack4/35
  Demux24/2 -> CAN FD Pack4/34
  Demux24/1 -> CAN FD Pack4/33
  TOS_AEB_LATOBJ/1 -> For Each Subsystem/1(In1)
  Demux1/2 -> CAN FD Pack1/2
  Demux1/1 -> CAN FD Pack1/1
  Demux1/3 -> CAN FD Pack1/3
  Demux1/4 -> CAN FD Pack1/4
  Demux1/5 -> CAN FD Pack1/5
  Demux1/6 -> CAN FD Pack1/6
  Demux1/7 -> CAN FD Pack1/7
  Demux1/8 -> CAN FD Pack1/8
  Demux1/9 -> CAN FD Pack1/9
  Demux1/10 -> CAN FD Pack1/10
  For Each Subsystem/1(FusionType) -> Demux1/1
  Demux2/1 -> CAN FD Pack1/11
  Demux2/2 -> CAN FD Pack1/12
  Demux2/3 -> CAN FD Pack1/13
  Demux2/4 -> CAN FD Pack1/14
  Demux2/5 -> CAN FD Pack1/15
  Demux2/6 -> CAN FD Pack1/16
  Demux2/7 -> CAN FD Pack1/17
  Demux2/8 -> CAN FD Pack1/18
  Demux2/9 -> CAN FD Pack1/19
  Demux2/10 -> CAN FD Pack1/20
  For Each Subsystem/2(ObjectID) -> Demux2/1  "ObjectID"
  Demux3/1 -> CAN FD Pack1/21
  Demux3/2 -> CAN FD Pack1/22
  Demux3/3 -> CAN FD Pack1/23
  Demux3/4 -> CAN FD Pack1/24
  Demux3/5 -> CAN FD Pack1/25
  Demux3/6 -> CAN FD Pack1/26
  Demux3/7 -> CAN FD Pack1/27
  Demux3/8 -> CAN FD Pack1/28
  Demux3/9 -> CAN FD Pack1/29
  Demux3/10 -> CAN FD Pack1/30
  For Each Subsystem/3(ObjectMovingOrientation) -> Demux3/1  "ObjectType"
  Demux4/1 -> CAN FD Pack1/31
  Demux4/2 -> CAN FD Pack1/32
  Demux4/3 -> CAN FD Pack1/33
  Demux4/4 -> CAN FD Pack1/34
  Demux4/5 -> CAN FD Pack1/35
  Demux4/6 -> CAN FD Pack1/36
  Demux4/7 -> CAN FD Pack1/37
  Demux4/8 -> CAN FD Pack1/38
  Demux4/9 -> CAN FD Pack1/39
  Demux4/10 -> CAN FD Pack1/40
  For Each Subsystem/4(ObjectMovingState) -> Demux4/1  "ObjectMovingState"
  Demux5/1 -> CAN FD Pack1/41
  Demux5/2 -> CAN FD Pack1/42
  Demux5/3 -> CAN FD Pack1/43
  Demux5/4 -> CAN FD Pack1/44
  Demux5/5 -> CAN FD Pack1/45
  Demux5/6 -> CAN FD Pack1/46
  Demux5/7 -> CAN FD Pack1/47
  Demux5/8 -> CAN FD Pack1/48
  Demux5/9 -> CAN FD Pack1/49
  Demux5/10 -> CAN FD Pack1/50
  For Each Subsystem/5(ObjectType) -> Demux5/1  "ObjectMovingOrientation"
  Demux6/1 -> CAN FD Pack1/51
  Demux6/2 -> CAN FD Pack1/52
  Demux6/3 -> CAN FD Pack1/53
  Demux6/4 -> CAN FD Pack1/54
  Demux6/5 -> CAN FD Pack1/55
  Demux6/6 -> CAN FD Pack1/56
  Demux6/7 -> CAN FD Pack1/57
  Demux6/8 -> CAN FD Pack1/58
  Demux6/9 -> CAN FD Pack1/59
  Demux6/10 -> CAN FD Pack1/60
  For Each Subsystem/6(dx) -> Demux6/1  "dx"
  Demux28/1 -> CAN FD Pack1/61
  Demux28/2 -> CAN FD Pack1/62
  Demux28/3 -> CAN FD Pack1/63
  Demux28/4 -> CAN FD Pack1/64
  Demux28/5 -> CAN FD Pack1/65
  Demux28/6 -> CAN FD Pack1/66
  Demux28/7 -> CAN FD Pack1/67
  Demux28/8 -> CAN FD Pack1/68
  Demux28/9 -> CAN FD Pack1/69
  Demux28/10 -> CAN FD Pack1/70
  For Each Subsystem/7(dy) -> Demux28/1  "dy"
